simulink model "DIME12_Ctrl_dSpaceHRBMAB"  (R2018b)
settings: Solver=ode1  StartTime=0.0  StopTime=inf  FixedStep=0.5  RelTol=1e-3
PostLoadFcn:
  | if any(exist('dsrtsu_mdlpostloadfcn', 'file') ~= 0), dsrtsu_mdlpostloadfcn('Execute', bdroot); end
InitFcn:
  | , if any(exist('dsmpb_private', 'file') ~= 0), dsmpb_private('dsmpb_mdlclblib', 'Init', bdroot); end,
  | load('LUT_PSM.mat')
  | load('Torque_ts.mat')
  | 
  | p = 1;
  | L_q = 1.575e-3;
  | L_d = L_q;
  | Psi_M = 0.0353*2*pi;
  | R_s = 639e-3;
  | Ts = 1/40e3;
  | J_ges = 9.56e-5;
  | d_viskos = 0.01;
  | mpsTestMaxVelocityDmd = 166.7;
  | mpsTestVelocityDmd = 0;
  | EDC_CURRENT_CONTROL_EXECUTION_PERIOD = 4e-5;
  | 
undefined symbols (not defined in the file or in its folder): d, motor_KF, Psidq, Psiqd, q, SimSampleT
libraries: simulink x37, dsmpblib x12, simulink_extras x3
(part 1 of 2)
PreSaveFcn:
  | , if any(exist('dsmpb_private', 'file') ~= 0), dsmpb_private('dsmpb_mdlclblib', 'PreSave', bdroot); end,
CloseFcn:
  | , if any(exist('dsmpb_private', 'file') ~= 0), dsmpb_private('dsmpb_mdlclblib', 'Close', bdroot); end,
settings Model: DSMPB_ID_DATA={'3134',struct('BlockId','04db4ddd-0369-4418-ae49-28ce71638d8c','SignalIds',{{'5c51ac2c-5fbb-4ba9-aa34-33d7867766ca','a6cd89eb-b981-47d6-bc47-5ca729bc3f45','097cfed2-f50c-4e25-bc62-441cc3621ec0'}}),'3136',struct('BlockId','3590bb54-d273-4af4-9544-5048f98a2daf','SignalIds',{{'c842c855-2857-45a6-a8e5-79953c06c9eb'}}),'3137',struct('BlockId','bccae625-1341-47c7-9337-55481b633b8f','SignalIds',{{'f61f6422-2fdc-4408-804f-4fad1389e9ca'}}),'3138',struct('BlockId','34b8a974-9a5d-46c5-a0f7-f433ccad648d','SignalIds',{{'09e6ef1a-8a88-4fa6-b01f-5871e321ecb2'}}),'3139',struct('BlockId','e0cdb478-2f16-48d9-bcde-88b35d629747','SignalIds',{{'a976c208-9896-475b-afed-9b9b9f9847b2','8f7e8e4e-2c4c-4faa-aa94-dc305397ccfc','84db2b89-11f0-4bb6-8049-e2d104c4d262'}}),'3140',struct('BlockId','fd95bb8a-93e4-455d-bc68-9a6da0afcd0d','SignalIds',{{'929c58ef-2907-4469-b920-2e801e504bc2'}}),'3142',struct('BlockId','72c4edce-58e5-47fd-a414-c19eae35a3a8','SignalIds',{{'d0a6c1a2-fd8d-466a-9efe-92e242699193'}}),'3223',struct('BlockId','5770f357-64e8-43e0-9a62-efd8e5c4a994','SignalIds',{{'84e8b84b-37b0-4755-b550-56b85c125762'}}),'3326',struct('BlockId','0213ed4f-146c-4d9a-827f-511852e41879','SignalIds',{{'cdea7f12-a251-4748-b247-1d592575f419'}}),'3327',struct('BlockId','ef935bd5-43af-450c-a12d-3eb1077517d5','SignalIds',{{'a65a6045-fefa-43b6-998f-670ac0cde20a'}}),'3328',struct('BlockId','6ee705ff-6fc1-4892-a215-acc4da7c45a2','SignalIds',{{'025f1da1-06c6-4956-b1e6-82a58301fd35'}}),'3342',struct('BlockId','89047cf2-e30b-4ee5-aefe-f8c97c394358','SignalIds',{{'983c3a74-9a59-4487-a442-b115395a8b56'}})}  RTICANMMDATA=struct('GeneralSetupData',struct('modelroot','C:\Jingyuan\DIME12_HRB\SimulinkModel','generalsettings',struct('filesettings',struct('destfolder',struct('Name','RTICANMM_FILES','Check',1),'buildfolder',struct('Name','.','Check',1),'AbsDestfolder',struct('Name','C:\Jingyuan\DIME12_HRB\SimulinkModel\RTICANMM_FILES'),'AbsBuildfolder',struct('Name','C:\Jingyuan\DIME12_HRB\SimulinkModel'))),'options',struct('addpaths',1,'rmpaths',1,'addtrcexclusion',true,'cannavigator',struct('checkmonitoring',0),'show_usrtrc',0,'use_usrtrc',0),'advanced',struct('options',ones(1,100)),'MPSetup',{{}},'RTI',struct('Type','DSRT','Ver','4.2','Date','02-Nov-2019'),'modelname','DIME12_Ctrl_dSpaceHRBMAB','block','DIME12_Ctrl_dSpaceHRBMAB'))  DSRTSU_INTERNAL_RTIFPGA=150  Creator=Z0185892  LastModifiedBy=Z644053
settings DataIOCC: ReturnWorkspaceOutputs=on
settings OptimizationCC: BlockReduction=off  ConditionallyExecuteInputs=off  OptimizeBlockIOStorage=off  BufferReuse=off  GlobalBufferReuse=off  ExpressionFolding=off  LocalBlockOutputs=off  OptimizeDataStoreBuffers=off  BusAssignmentInplaceUpdate=off
settings DebuggingCC: TasksWithSamePriorityMsg=none  UnconnectedInputMsg=none  UnconnectedOutputMsg=none
settings HardwareCC: ProdBitPerPointer=32  ProdBitPerSizeT=32  ProdBitPerPtrDiffT=32  ProdLargestAtomicInteger=Integer  ProdWordSize=32  ProdHWDeviceType=Custom Processor->Custom
settings SFSimCC: MATLABDynamicMemAlloc=off
settings RTWCC: SystemTargetFile=dsrt.tlc  GenCodeOnly=on  MakeCommand=make_dsrt  TemplateMakefile=dsrt_default_tmf  Description=dSPACE Run-Time Target (for VEOS on Windows and ConfigurationDesk)  RTWVerbose=off
settings STFCustomTargetCC: TargetLangStandard=C99 (ISO)  ParMdlRefBuildCompliant=on  SystemTargetFile=dsrt.tlc
settings GRTTargetCC: CompOptLevelCompliant=off  ConcurrentExecutionCompliant=off  CombineOutputUpdateFcns=off  MatFileLogging=off  CPPClassGenCompliant=off  UseToolchainInfoCompliant=off

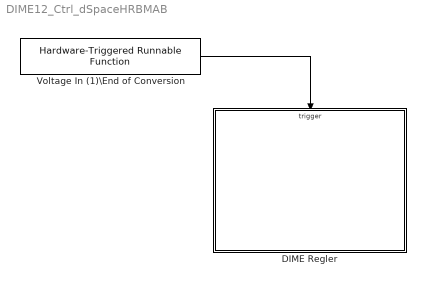
== system DIME12_Ctrl_dSpaceHRBMAB ==
  DIME Regler : Subsystem
  Voltage In (1)\End of Conversion : dsmpblib/Hardware-Triggered Runnable Function
      settings: SourceProductName=dSPACE Model Interface Blockset
  wires:
  Voltage In (1)\End of Conversion/1 -> DIME Regler/Trigger

== system DIME12_Ctrl_dSpaceHRBMAB/DIME Regler ==
  Trigger : TriggerPort  TriggerType=function-call  VariantControl=Variant  PortDimensions=1
  Bus Selector : BusSelector  OutputSignals=Omega_rps,Iphase1,Iphase2,Iphase3,Temperature
  Controller : Subsystem
  Gain : Gain  Gain=pi/30
  Outputs : Subsystem
  TqDmd : Constant  Value=2
  Velocity_RPM : Constant  Value=1000
  dSpace Measurement : Subsystem
  wires:
  TqDmd/1 -> Controller/1(TorqueDmd)
  Velocity_RPM/1 -> Gain/1
  Gain/1 -> Controller/2(VelocityDmd)
  dSpace Measurement/1(Bus Measurements) -> Bus Selector/1, Controller/3(Bus_measurements)
  Controller/1(u_alpha_beta_voltage_dmd) -> Outputs/1(AlphaBetaVoltage)
  Bus Selector/1 -> Outputs/2(meclVelocityMAB)  "<Omega_rps>"
  Bus Selector/2 -> Outputs/3(IPhase1)  "<Iphase1>"
  Bus Selector/3 -> Outputs/4(IPhase2)  "<Iphase2>"
  Bus Selector/4 -> Outputs/5(IPhase3)  "<Iphase3>"
  Bus Selector/5 -> Outputs/6(Temperature)  "<Temperature>"

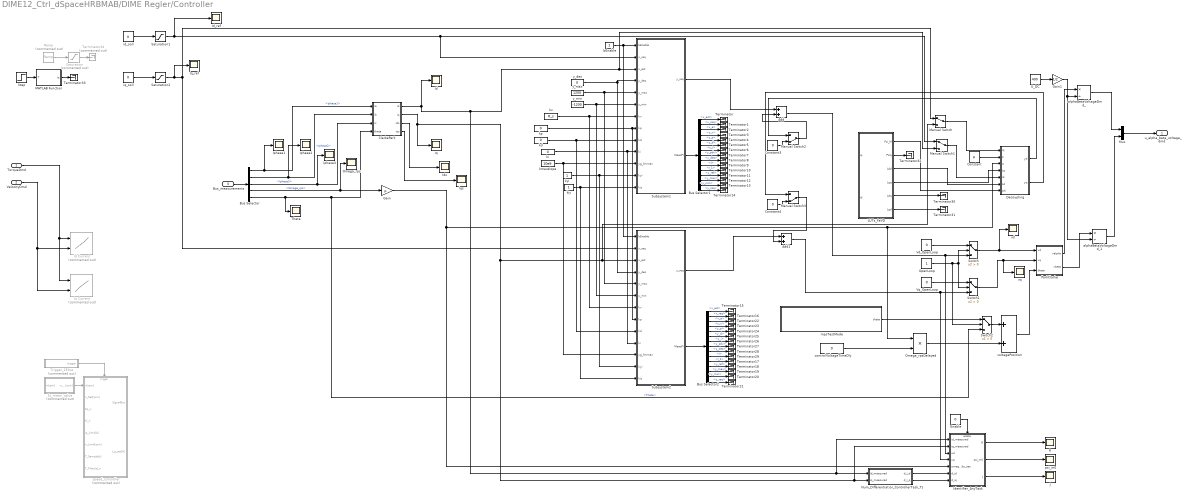
== system DIME12_Ctrl_dSpaceHRBMAB/DIME Regler/Controller ==
  TorqueDmd : Inport
  VelocityDmd : Inport  Port=2
  Bus_measurements : Inport  Port=3
  5x_mean_value : Subsystem  Commented=on
  Add : Sum
  Add1 : Sum
  Bus Selector : BusSelector  OutputSignals=Iphase1,Iphase2,Iphase3,Omega_rps,Theta
  Bus Selector1 : BusSelector  OutputSignals=x_act,x_req,x_e,y_v,y_p,y_d,y_i,y_pdv,y_des,I,I_1,y_ref,y_max,y_min,y_req
  Bus Selector2 : BusSelector  OutputSignals=x_act,x_req,x_e,y_v,y_p,y_d,y_i,y_pdv,y_des,I,I_1,y_ref,y_max,y_min,y_req
  ClarkePark : MATLAB Function  TreatAsAtomicUnit=on
  Constant : Constant  Value=p
  Constant3 : Constant  Value=0
  Constant4 : Constant  Value=0
  Decoupling : MATLAB Function  TreatAsAtomicUnit=on
  Enable : Constant  Value=0
  Gain : Gain  Gain=p
  Gain1 : Gain  Gain=1/2
  Id : Scope
  Id Current : Lookup_n-D  Commented=on  BreakpointsForDimension1=motor_KF.motTorqueDmd  BreakpointsForDimension2=motor_KF.motAbsltMeclVelocity  Table=motor_KF.idcurrent  InternalRulePriority=Speed  RndMeth=Simplest  InputSameDT=on
  Id_ref : Scope
  Identifier_AnyTask : Subsystem
  Ids : Scope
  Iphase1 : Scope
  Iphase2 : Scope
  Iphase3 : Scope
  Iq : Scope
  Iq Current : Lookup_n-D  Commented=on  BreakpointsForDimension1=motor_KF.motTorqueDmd  BreakpointsForDimension2=motor_KF.motAbsltMeclVelocity  Table=motor_KF.iqcurrent  InternalRulePriority=Speed  RndMeth=Simplest  InputSameDT=on
  Iq_ref : Scope
  Iqs : Scope
  J : Scope
  LUTs_FeVD : Subsystem
  MATLAB Function : MATLAB Function  TreatAsAtomicUnit=on
  Manual Switch : ManualSwitch
  Manual Switch1 : ManualSwitch
  Manual Switch2 : ManualSwitch  CurrentSetting=0
  Manual Switch3 : ManualSwitch  CurrentSetting=0
  Mux : Mux  Inputs=2
  Num_Differentiatior_ControllerTask_Ts : Subsystem
  Omega_rps : Scope
  Omega_rpsDelayed : Product  Inputs=**  RndMeth=Zero
  OpenLoop : Constant
  ParkClarke : MATLAB Function  TreatAsAtomicUnit=on
  R : Scope
  Ramp : simulink/Sources/Ramp  Commented=on  slope=1  start=0  InitialOutput=0
  Saturation : Saturate  Commented=on  UpperLimit=15  LowerLimit=0
  Saturation1 : Saturate  UpperLimit=18  LowerLimit=-18  LinearizeAsGain=off
  Saturation2 : Saturate  UpperLimit=18  LowerLimit=0  LinearizeAsGain=off
  Step : Step  Time=0.05  After=0
  Subsystem1 : Subsystem
  Subsystem2 : Subsystem
  Switch : Switch  Criteria=u2 > Threshold
  Switch1 : Switch  Criteria=u2 > Threshold
  Switch2 : Switch  Criteria=u2 > Threshold
  Terminator{,1..33} (34 alike) : Terminator
  Terminator34 : Terminator  Commented=on
  Theta : Scope
  Trigger_250us : Subsystem  Commented=on
  U_DC : Constant  Value=400
  Vd_OpenLoop : Constant  Value=0
  Vq_OpenLoop : Constant  Value=0
  alphaBetaVoltageDmd_ : Product  Inputs=*/  RndMeth=Zero
  alphaBetaVoltageDmd_1 : Product  Inputs=*/  RndMeth=Zero
  bEnable : Constant
  controlVoltageTimeDly : Constant  LoadFcn=|  Value=0  SampleTime=-1
      | if exist('SL_HighlightBlocks', 'file') == 2
      |     if ~SL_HighlightBlocks(gcb, [])
      |         warning(['Unable to set properties for ' gcb])
      |     end
      | end
      settings: AttributesFormatString=Changed: SampleTime
  id_soll : Constant  Value=0
  iq_soll : Constant  Value=0
  kd : Constant  Value=0
  ki : Constant  Value=0
  kiy : Constant
  kmaxslope : Constant  Value=10e9
  kp : Constant  Value=0
  kv : Constant  Value=R_s
  kyi : Constant
  mpsTestMode : Subsystem
  psi_m0 : Scope
  speed_controller : Subsystem  Commented=on
  vd : Scope
  voltagePosition : Sum
  vq : Scope
  y_des : Constant  Value=0
  y_max : Constant  Value=1200
  y_min : Constant  Value=-1200
  u_alpha_beta_voltage_dmd : Outport  VectorParamsAs1DForOutWhenUnconnected=on
  wires:
  TorqueDmd/1 -> Iq Current/1, Id Current/1
  VelocityDmd/1 -> Iq Current/2, Id Current/2
  Bus Selector/2 -> Iphase2/1, ClarkePark/2(ib)  "<Iphase2>"
  Bus Selector/1 -> Iphase1/1, ClarkePark/1(ia)  "<Iphase1>"
  Bus Selector/3 -> Iphase3/1, ClarkePark/3(ic)  "<Iphase3>"
  Bus_measurements/1 -> Bus Selector/1
  Bus Selector/4 -> Gain/1, Omega_rps/1  "<Omega_rps>"
  Bus Selector1/9 -> Terminator8/1  "<y_des>"
  Bus Selector1/6 -> Terminator5/1  "<y_d>"
  Bus Selector1/12 -> Terminator11/1  "<y_ref>"
  Bus Selector1/15 -> Terminator14/1  "<y_req>"
  kp/1 -> Subsystem2/8(kp), Subsystem1/8(kp)
  Bus Selector1/4 -> Terminator3/1  "<y_v>"
  Bus Selector1/5 -> Terminator4/1  "<y_p>"
  Bus Selector1/2 -> Terminator1/1  "<x_req>"
  Bus Selector1/13 -> Terminator12/1  "<y_max>"
  kd/1 -> Subsystem2/9(kd), Subsystem1/9(kd)
  Bus Selector1/8 -> Terminator7/1  "<y_pdv>"
  Bus Selector1/10 -> Terminator9/1  "<I>"
  Subsystem1/2(MeasPi) -> Bus Selector1/1
  Bus Selector1/7 -> Terminator6/1  "<y_i>"
  Bus Selector1/1 -> Terminator/1  "<x_act>"
  Bus Selector1/14 -> Terminator13/1  "<y_min>"
  Bus Selector1/11 -> Terminator10/1  "<I_1>"
  Bus Selector1/3 -> Terminator2/1  "<x_e>"
  Bus Selector2/9 -> Terminator28/1  "<y_des>"
  y_des/1 -> Subsystem1/4(y_des), Subsystem2/4(y_des)
  kmaxslope/1 -> Subsystem2/11(yg_limmax), Subsystem1/11(yg_limmax)
  kiy/1 -> Subsystem2/13(kiy), Subsystem1/13(kiy)
  y_max/1 -> Subsystem2/5(y_max), Subsystem1/5(y_max)
  Bus Selector2/6 -> Terminator25/1  "<y_d>"
  Bus Selector2/12 -> Terminator18/1  "<y_ref>"
  y_min/1 -> Subsystem2/6(y_min), Subsystem1/6(y_min)
  Bus Selector2/15 -> Terminator21/1  "<y_req>"
  Bus Selector2/4 -> Terminator23/1  "<y_v>"
  Bus Selector2/5 -> Terminator24/1  "<y_p>"
  Bus Selector2/2 -> Terminator16/1  "<x_req>"
  Bus Selector2/13 -> Terminator19/1  "<y_max>"
  ki/1 -> Subsystem2/10(ki), Subsystem1/10(ki)
  kyi/1 -> Subsystem1/12(kyi), Subsystem2/12(kyi)
  kv/1 -> Subsystem2/7(kv), Subsystem1/7(kv)
  Bus Selector2/8 -> Terminator27/1  "<y_pdv>"
  Bus Selector2/10 -> Terminator29/1  "<I>"
  Subsystem2/2(MeasPi) -> Bus Selector2/1
  Bus Selector2/7 -> Terminator26/1  "<y_i>"
  Bus Selector2/1 -> Terminator15/1  "<x_act>"
  Bus Selector2/14 -> Terminator20/1  "<y_min>"
  Bus Selector2/11 -> Terminator17/1  "<I_1>"
  Bus Selector2/3 -> Terminator22/1  "<x_e>"
  bEnable/1 -> Subsystem2/1(bEnable), Subsystem1/1(bEnable)
  ClarkePark/1(id) -> Identifier_AnyTask/1(id_measured), Num_Differentiatior_ControllerTask_Ts/1(id_measured), Manual Switch1/2, Subsystem1/3(x_act), Id/1
  ClarkePark/2(iq) -> Iq/1, Identifier_AnyTask/2(iq_measured), Num_Differentiatior_ControllerTask_Ts/2(iq_measured), Manual Switch/2, Subsystem2/3(x_act)
  Subsystem1/1(y_req) -> Add/1
  Decoupling/1(yd) -> Manual Switch2/1
  Subsystem2/1(y_req) -> Add1/1
  Decoupling/2(yq) -> Manual Switch3/1
  Add1/1 -> Identifier_AnyTask/4(uq), Switch1/3
  Add/1 -> Identifier_AnyTask/3(ud), Switch/3
  LUTs_FeVD/6(Lqd) -> Terminator31/1
  LUTs_FeVD/5(Ldq) -> Terminator30/1
  LUTs_FeVD/3(Ldd) -> Decoupling/6(Ld)
  LUTs_FeVD/4(Lqq) -> Decoupling/4(Lq)
  LUTs_FeVD/1(Psi_M) -> Decoupling/7(phi)
  Constant/1 -> Decoupling/2(p)
  Gain/1 -> Identifier_AnyTask/5(omega_elec_1by_sec), Omega_rpsDelayed/1, Decoupling/3(w)
  LUTs_FeVD/2(Psiq) -> Terminator32/1
  ParkClarke/1(valpha) -> alphaBetaVoltageDmd_/1
  U_DC/1 -> Gain1/1
  ParkClarke/2(vbeta) -> alphaBetaVoltageDmd_1/1
  alphaBetaVoltageDmd_/1 -> Mux/1
  alphaBetaVoltageDmd_1/1 -> Mux/2
  Mux/1 -> u_alpha_beta_voltage_dmd/1
  id_soll/1 -> Saturation1/1
  iq_soll/1 -> Saturation2/1
  Manual Switch/1 -> Decoupling/1(iq)
  Manual Switch1/1 -> Decoupling/5(id)
  Constant3/1 -> Manual Switch2/2
  Manual Switch2/1 -> Add/2
  Constant4/1 -> Manual Switch3/2
  Manual Switch3/1 -> Add1/2
  Step/1 -> MATLAB Function/1(T)
  Bus Selector/5 -> Theta/1, Switch2/3, ClarkePark/4(theta)  "<Theta>"
  Vd_OpenLoop/1 -> Switch/1
  Switch/1 -> vd/1, ParkClarke/1(vd)
  Vq_OpenLoop/1 -> Switch1/1
  Switch1/1 -> vq/1, ParkClarke/2(vq)
  mpsTestMode/1(theta) -> Switch2/1
  OpenLoop/1 -> Switch2/2, Switch/2, Switch1/2
  Switch2/1 -> voltagePosition/1
  MATLAB Function/1(iq) -> Terminator33/1
  controlVoltageTimeDly/1 -> Omega_rpsDelayed/2
  Omega_rpsDelayed/1 -> voltagePosition/2
  voltagePosition/1 -> ParkClarke/3(theta)
  Ramp/1 -> Saturation/1
  Saturation/1 -> Terminator34/1
  Saturation1/1 -> Id_ref/1, Manual Switch1/1, Subsystem1/2(x_req)
  Saturation2/1 -> Iq_ref/1, Manual Switch/1, Subsystem2/2(x_req)
  ClarkePark/3(ids) -> Ids/1
  ClarkePark/4(iqs) -> Iqs/1
  Num_Differentiatior_ControllerTask_Ts/1(d_i_d) -> Identifier_AnyTask/6(d_id)
  Identifier_AnyTask/2(psi_m0) -> psi_m0/1
  Identifier_AnyTask/3(J) -> J/1
  Num_Differentiatior_ControllerTask_Ts/2(d_i_q) -> Identifier_AnyTask/7(d_iq)
  Identifier_AnyTask/1(R) -> R/1
  Enable/1 -> Identifier_AnyTask/Enable
  Gain1/1 -> alphaBetaVoltageDmd_/2, alphaBetaVoltageDmd_1/2
  5x_mean_value/1(n_mean[rpm]) -> speed_controller/1(n[rpm])
  Trigger_250us/1(trigger) -> speed_controller/Trigger

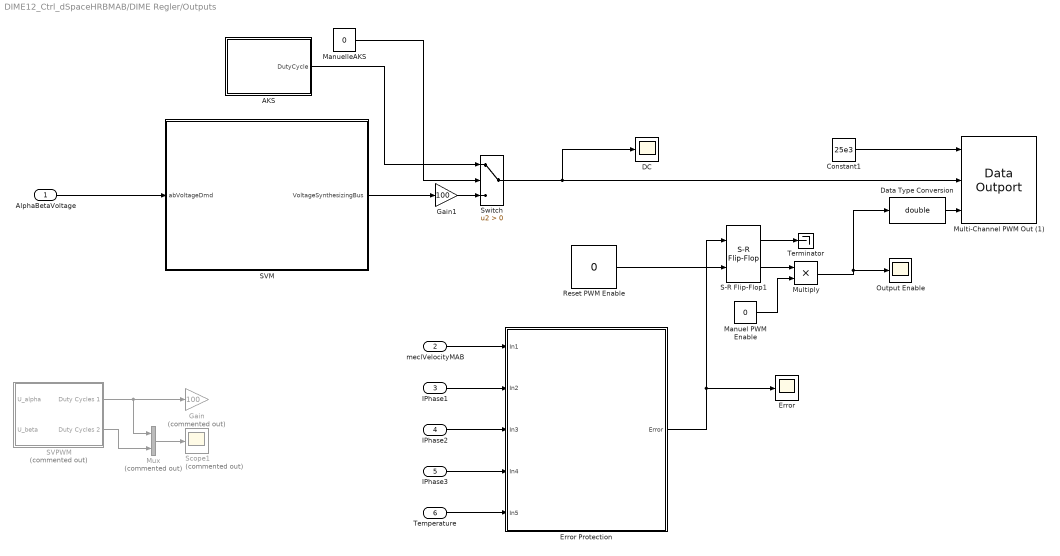
== system DIME12_Ctrl_dSpaceHRBMAB/DIME Regler/Outputs ==
  AlphaBetaVoltage : Inport
  meclVelocityMAB : Inport  Port=2
  IPhase1 : Inport  Port=3
  IPhase2 : Inport  Port=4
  IPhase3 : Inport  Port=5
  Temperature : Inport  Port=6
  AKS : Subsystem
  Constant1 : Constant  Value=25e3
  DC : Scope
  Data Type Conversion : DataTypeConversion  OutDataTypeStr=double
  Error : Scope
  Error Protection : Subsystem
  Gain : Gain  Commented=on  Gain=100
  Gain1 : Gain  Gain=100
  Manuel PWM Enable : Constant  Value=0
  ManuelleAKS : Constant  Value=0
  Multi-Channel PWM Out (1) : dsmpblib/Data Outport  Priority=-10000
      settings: SourceProductName=dSPACE Model Interface Blockset
  Multiply : Product
  Mux : Mux  Commented=on  Inputs=2
  Output Enable : Scope
  Reset PWM Enable : Constant  Value=0  OutDataTypeStr=Inherit: Inherit via back propagation
  S-R Flip-Flop1 : simulink_extras/Flip Flops/S-R Flip-Flop  initial_condition=1
  SVM : Subsystem  VariantControl=Variant
  SVPWM : Subsystem  Commented=on
  Scope1 : Scope  Commented=on
  Switch : Switch  Criteria=u2 > Threshold
  Terminator : Terminator
  wires:
  Constant1/1 -> Multi-Channel PWM Out (1)/1
  SVPWM/2(Duty Cycles 2) -> Mux/2
  SVPWM/1(Duty Cycles 1) -> Mux/1, Gain/1
  Mux/1 -> Scope1/1
  AlphaBetaVoltage/1 -> SVM/1(abVoltageDmd)
  SVM/1(VoltageSynthesizingBus) -> Gain1/1
  AKS/1(DutyCycle) -> Switch/1
  ManuelleAKS/1 -> Switch/2
  Gain1/1 -> Switch/3
  Reset PWM Enable/1 -> S-R Flip-Flop1/2
  meclVelocityMAB/1 -> Error Protection/1(In1)
  IPhase1/1 -> Error Protection/2(In2)
  IPhase2/1 -> Error Protection/3(In3)
  IPhase3/1 -> Error Protection/4(In4)
  Temperature/1 -> Error Protection/5(In5)
  Error Protection/1(Error) -> S-R Flip-Flop1/1, Error/1
  S-R Flip-Flop1/1 -> Terminator/1
  Data Type Conversion/1 -> Multi-Channel PWM Out (1)/3
  S-R Flip-Flop1/2 -> Multiply/1
  Manuel PWM Enable/1 -> Multiply/2
  Multiply/1 -> Output Enable/1, Data Type Conversion/1
  Switch/1 -> Multi-Channel PWM Out (1)/2, DC/1

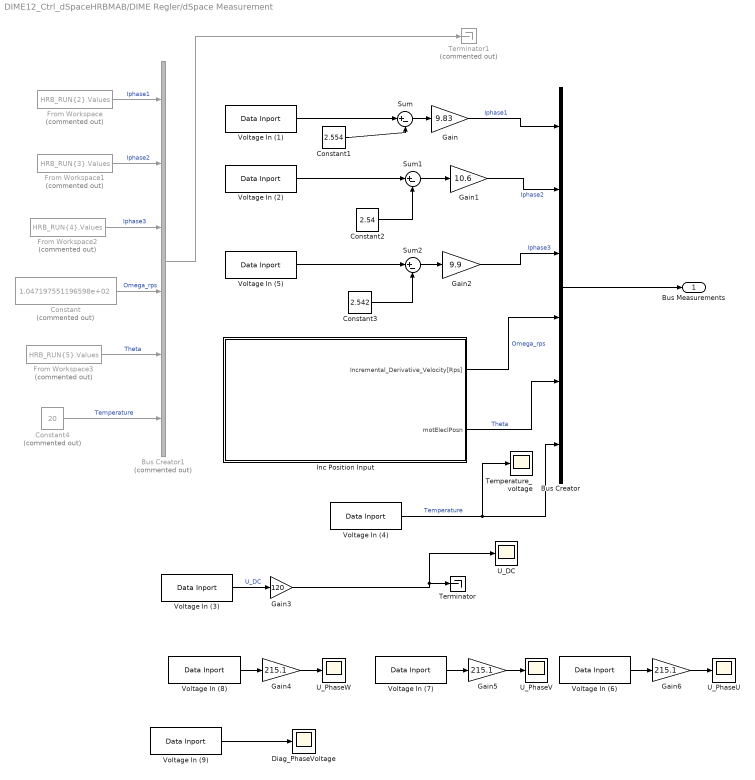
== system DIME12_Ctrl_dSpaceHRBMAB/DIME Regler/dSpace Measurement ==
  Bus Creator : BusCreator  Inputs=6
  Bus Creator1 : BusCreator  Commented=on  Inputs=6
  Constant : Constant  Commented=on  Value=1.047197551196598e+02  SampleTime=-1
  Constant1 : Constant  Value=2.554
  Constant2 : Constant  Value=2.54
  Constant3 : Constant  Value=2.542
  Constant4 : Constant  Commented=on  Value=20  SampleTime=-1
  Diag_PhaseVoltage : Scope
  From Workspace : FromWorkspace  Commented=on  VariableName=HRB_RUN{2}.Values
  From Workspace1 : FromWorkspace  Commented=on  VariableName=HRB_RUN{3}.Values
  From Workspace2 : FromWorkspace  Commented=on  VariableName=HRB_RUN{4}.Values
  From Workspace3 : FromWorkspace  Commented=on  VariableName=HRB_RUN{5}.Values
  Gain : Gain  Gain=9.83
  Gain1 : Gain  Gain=10.6
  Gain2 : Gain  Gain=9.9
  Gain3 : Gain  Gain=120
  Gain4 : Gain  Gain=215.1
  Gain5 : Gain  Gain=215.1
  Gain6 : Gain  Gain=215.1
  Inc Position Input : Subsystem
  Sum : Sum  Inputs=|+-
  Sum1 : Sum  Inputs=|+-
  Sum2 : Sum  Inputs=|+-
  Temperature_voltage : Scope
  Terminator : Terminator
  Terminator1 : Terminator  Commented=on
  U_DC : Scope
  U_PhaseU : Scope
  U_PhaseV : Scope
  U_PhaseW : Scope
  Voltage In (1) : dsmpblib/Data Inport  Priority=10000
      settings: SourceProductName=dSPACE Model Interface Blockset
  Voltage In (2) : dsmpblib/Data Inport  Priority=10000
      settings: SourceProductName=dSPACE Model Interface Blockset
  Voltage In (3) : dsmpblib/Data Inport  Priority=10000
      settings: SourceProductName=dSPACE Model Interface Blockset
  Voltage In (4) : dsmpblib/Data Inport  Priority=10000
      settings: SourceProductName=dSPACE Model Interface Blockset
  Voltage In (5) : dsmpblib/Data Inport  Priority=10000
      settings: SourceProductName=dSPACE Model Interface Blockset
  Voltage In (6) : dsmpblib/Data Inport  Priority=10000
      settings: SourceProductName=dSPACE Model Interface Blockset
  Voltage In (7) : dsmpblib/Data Inport  Priority=10000
      settings: SourceProductName=dSPACE Model Interface Blockset
  Voltage In (8) : dsmpblib/Data Inport  Priority=10000
      settings: SourceProductName=dSPACE Model Interface Blockset
  Voltage In (9) : dsmpblib/Data Inport  Priority=10000
      settings: SourceProductName=dSPACE Model Interface Blockset
  Bus Measurements : Outport
  wires:
  Constant2/1 -> Sum1/2
  Sum1/1 -> Gain1/1
  Gain1/1 -> Bus Creator/2  "Iphase2"
  Voltage In (1)/1 -> Sum/1
  Voltage In (5)/1 -> Sum2/1
  Gain/1 -> Bus Creator/1  "Iphase1"
  Sum2/1 -> Gain2/1
  Voltage In (2)/1 -> Sum1/1
  Constant1/1 -> Sum/2
  Gain2/1 -> Bus Creator/3  "Iphase3"
  Constant3/1 -> Sum2/2
  Sum/1 -> Gain/1
  Inc Position Input/1(Incremental_Derivative_Velocity[Rps]) -> Bus Creator/4  "Omega_rps"
  Inc Position Input/2(motEleclPosn) -> Bus Creator/5  "Theta"
  Voltage In (4)/1 -> Temperature_voltage/1, Bus Creator/6  "Temperature"
  From Workspace2/1 -> Bus Creator1/3  "Iphase3"
  From Workspace3/1 -> Bus Creator1/5  "Theta"
  Constant/1 -> Bus Creator1/4  "Omega_rps"
  Constant4/1 -> Bus Creator1/6  "Temperature"
  Voltage In (3)/1 -> Gain3/1  "U_DC"
  Gain3/1 -> U_DC/1, Terminator/1
  From Workspace/1 -> Bus Creator1/1  "Iphase1"
  From Workspace1/1 -> Bus Creator1/2  "Iphase2"
  Bus Creator1/1 -> Terminator1/1
  Bus Creator/1 -> Bus Measurements/1
  Voltage In (8)/1 -> Gain4/1
  Voltage In (7)/1 -> Gain5/1
  Voltage In (6)/1 -> Gain6/1
  Gain4/1 -> U_PhaseW/1
  Gain5/1 -> U_PhaseV/1
  Gain6/1 -> U_PhaseU/1
  Voltage In (9)/1 -> Diag_PhaseVoltage/1

== system DIME12_Ctrl_dSpaceHRBMAB/DIME Regler/Controller/5x_mean_value ==
  n[rpm] : Inport
  Gain : Gain  Gain=1/5
  Memory{,1..3} (4 alike) : Memory  InheritSampleTime=on
  Sum : Sum  Inputs=+++++
  n_mean[rpm] : Outport
  wires:
  n[rpm]/1 -> Sum/1, Memory/1
  Memory/1 -> Sum/2, Memory1/1
  Memory1/1 -> Sum/3, Memory2/1
  Memory2/1 -> Sum/4, Memory3/1
  Memory3/1 -> Sum/5
  Sum/1 -> Gain/1
  Gain/1 -> n_mean[rpm]/1

== system DIME12_Ctrl_dSpaceHRBMAB/DIME Regler/Controller/Identifier_AnyTask ==
  id_measured : Inport
  iq_measured : Inport  Port=2
  ud : Inport  Port=3
  uq : Inport  Port=4
  omega_elec_1by_sec : Inport  Port=5
  d_id : Inport  Port=6
  d_iq : Inport  Port=7
  Enable : EnablePort  StatesWhenEnabling=reset
  NN Identifier : MATLAB Function  TreatAsAtomicUnit=on
  StepsizeIntegrator : Constant  Value=1e-4
  gains : Constant  Value=1e-3
  psim0_est : Constant  Value=0.1
  takeover : Constant  Value=0
  R : Outport  VectorParamsAs1DForOutWhenUnconnected=on
  psi_m0 : Outport  Port=2  VectorParamsAs1DForOutWhenUnconnected=on
  J : Outport  Port=3  VectorParamsAs1DForOutWhenUnconnected=on
  wires:
  id_measured/1 -> NN Identifier/2(id)
  StepsizeIntegrator/1 -> NN Identifier/1(h)
  gains/1 -> NN Identifier/12(Gamma_W_psi), NN Identifier/11(Gamma_Theta_psi), NN Identifier/10(Gamma_W_R), NN Identifier/9(Gamma_Theta_R)
  NN Identifier/2(psi_m0) -> psi_m0/1
  NN Identifier/1(R) -> R/1
  NN Identifier/3(J) -> J/1
  uq/1 -> NN Identifier/5(uq)
  omega_elec_1by_sec/1 -> NN Identifier/6(omega)
  ud/1 -> NN Identifier/4(ud)
  iq_measured/1 -> NN Identifier/3(iq)
  d_id/1 -> NN Identifier/7(d_id)
  d_iq/1 -> NN Identifier/8(d_iq)
  takeover/1 -> NN Identifier/13(takeover)
  psim0_est/1 -> NN Identifier/14(psim0_est)

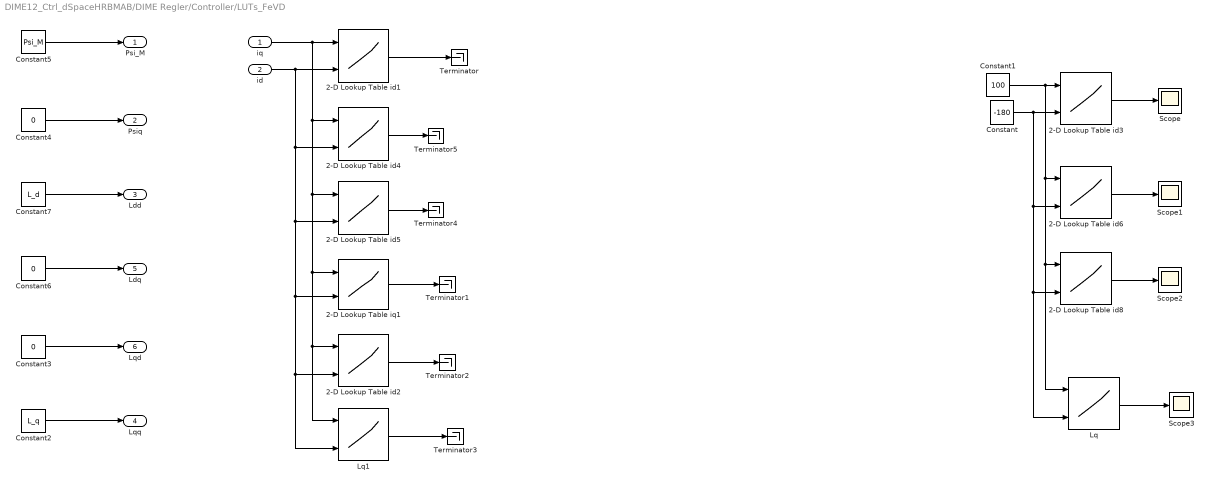
== system DIME12_Ctrl_dSpaceHRBMAB/DIME Regler/Controller/LUTs_FeVD ==
  iq : Inport
  id : Inport  Port=2
  2-D Lookup Table id1 : Lookup_n-D  BreakpointsForDimension1=|  BreakpointsForDimension2=|  Table=motor_KF.Psi_d'  InternalRulePriority=Speed  RndMeth=Simplest  InputSameDT=on
      BreakpointsForDimension2=|
      | [-220
      | -200
      | -180
      | -160
      | -140
      | -120
      | -100
      | -80
      | -60
      | -40
      | -20
      | 0
      | ]
      BreakpointsForDimension1=|
      | [0	20	40	60	80	100	120	140	160	180	200	220
      | ]
  2-D Lookup Table id2 : Lookup_n-D  BreakpointsForDimension1=q  BreakpointsForDimension2=d  Table=Psiqd  InternalRulePriority=Speed  RndMeth=Simplest  InputSameDT=on
  2-D Lookup Table id3 : Lookup_n-D  BreakpointsForDimension1=|  BreakpointsForDimension2=|  Table=motor_KF.Psi_d'  InternalRulePriority=Speed  RndMeth=Simplest  InputSameDT=on
      BreakpointsForDimension2=|
      | [-220
      | -200
      | -180
      | -160
      | -140
      | -120
      | -100
      | -80
      | -60
      | -40
      | -20
      | 0
      | ]
      BreakpointsForDimension1=|
      | [0	20	40	60	80	100	120	140	160	180	200	220
      | ]
  2-D Lookup Table id4 : Lookup_n-D  BreakpointsForDimension1=motor_KF.iqgrid  BreakpointsForDimension2=motor_KF.idgrid  Table=motor_KF.Psi_q'  InternalRulePriority=Speed  RndMeth=Simplest  InputSameDT=on
  2-D Lookup Table id5 : Lookup_n-D  BreakpointsForDimension1=motor_KF.iqgrid  BreakpointsForDimension2=motor_KF.idgrid  Table=motor_KF.Ld'  InternalRulePriority=Speed  RndMeth=Simplest  InputSameDT=on
  2-D Lookup Table id6 : Lookup_n-D  BreakpointsForDimension1=motor_KF.iqgrid  BreakpointsForDimension2=motor_KF.idgrid  Table=motor_KF.Psi_q'  InternalRulePriority=Speed  RndMeth=Simplest  InputSameDT=on
  2-D Lookup Table id8 : Lookup_n-D  BreakpointsForDimension1=motor_KF.iqgrid  BreakpointsForDimension2=motor_KF.idgrid  Table=motor_KF.Ld'  InternalRulePriority=Speed  RndMeth=Simplest  InputSameDT=on
  2-D Lookup Table iq1 : Lookup_n-D  BreakpointsForDimension1=q  BreakpointsForDimension2=d  Table=Psidq  InternalRulePriority=Speed  RndMeth=Simplest  InputSameDT=on
  Constant : Constant  Value=-180
  Constant1 : Constant  Value=100
  Constant2 : Constant  Value=L_q
  Constant3 : Constant  Value=0
  Constant4 : Constant  Value=0
  Constant5 : Constant  Value=Psi_M
  Constant6 : Constant  Value=0
  Constant7 : Constant  Value=L_d
  Lq : Lookup_n-D  BreakpointsForDimension1=motor_KF.iqgrid  BreakpointsForDimension2=motor_KF.idgrid  Table=motor_KF.Lq'  InternalRulePriority=Speed  RndMeth=Simplest  InputSameDT=on
  Lq1 : Lookup_n-D  BreakpointsForDimension1=motor_KF.iqgrid  BreakpointsForDimension2=motor_KF.idgrid  Table=motor_KF.Lq'  InternalRulePriority=Speed  RndMeth=Simplest  InputSameDT=on
  Scope{,1..3} (4 alike) : Scope
  Terminator{,1..5} (6 alike) : Terminator
  Psi_M : Outport  VectorParamsAs1DForOutWhenUnconnected=on
  Psiq : Outport  Port=2  VectorParamsAs1DForOutWhenUnconnected=on
  Ldd : Outport  Port=3  VectorParamsAs1DForOutWhenUnconnected=on
  Lqq : Outport  Port=4  VectorParamsAs1DForOutWhenUnconnected=on
  Ldq : Outport  Port=5  VectorParamsAs1DForOutWhenUnconnected=on
  Lqd : Outport  Port=6  VectorParamsAs1DForOutWhenUnconnected=on
  wires:
  iq/1 -> 2-D Lookup Table id1/1, 2-D Lookup Table id4/1, 2-D Lookup Table id5/1, Lq1/1, 2-D Lookup Table id2/1, 2-D Lookup Table iq1/1
  id/1 -> 2-D Lookup Table id1/2, 2-D Lookup Table id4/2, 2-D Lookup Table id5/2, Lq1/2, 2-D Lookup Table id2/2, 2-D Lookup Table iq1/2
  2-D Lookup Table id3/1 -> Scope/1
  Constant1/1 -> Lq/1, 2-D Lookup Table id8/1, 2-D Lookup Table id6/1, 2-D Lookup Table id3/1
  Constant/1 -> Lq/2, 2-D Lookup Table id8/2, 2-D Lookup Table id6/2, 2-D Lookup Table id3/2
  2-D Lookup Table id6/1 -> Scope1/1
  Lq/1 -> Scope3/1
  2-D Lookup Table id8/1 -> Scope2/1
  Constant4/1 -> Psiq/1
  Constant5/1 -> Psi_M/1
  Constant3/1 -> Lqd/1
  Constant7/1 -> Ldd/1
  Constant2/1 -> Lqq/1
  Constant6/1 -> Ldq/1
  2-D Lookup Table id1/1 -> Terminator/1
  Lq1/1 -> Terminator3/1
  2-D Lookup Table id2/1 -> Terminator2/1
  2-D Lookup Table iq1/1 -> Terminator1/1
  2-D Lookup Table id5/1 -> Terminator4/1
  2-D Lookup Table id4/1 -> Terminator5/1

== system DIME12_Ctrl_dSpaceHRBMAB/DIME Regler/Controller/Num_Differentiatior_ControllerTask_Ts ==
  id_measured : Inport
  iq_measured : Inport  Port=2
  Diff_Gain : Gain  Gain=5e3
  Diff_Gain2 : Gain  Gain=5e3
  Int : Subsystem
  Int1 : Subsystem
  Sum : Sum  Inputs=|+-
  Sum1 : Sum  Inputs=|+-
  compare_id : Scope  NumInputPorts=2
  compare_iq : Scope  NumInputPorts=2
  d_i_d : Outport  VectorParamsAs1DForOutWhenUnconnected=on
  d_i_q : Outport  Port=2  VectorParamsAs1DForOutWhenUnconnected=on
  wires:
  Sum/1 -> Diff_Gain/1
  Diff_Gain2/1 -> d_i_q/1, Int1/1(i_q_p)
  Diff_Gain/1 -> d_i_d/1, Int/1(i_d_p)
  Int/1(i_d) -> compare_id/2, Sum/2  "id"
  Sum1/1 -> Diff_Gain2/1
  Int1/1(i_q) -> compare_iq/2, Sum1/2  "iq"
  id_measured/1 -> compare_id/1, Sum/1
  iq_measured/1 -> compare_iq/1, Sum1/1

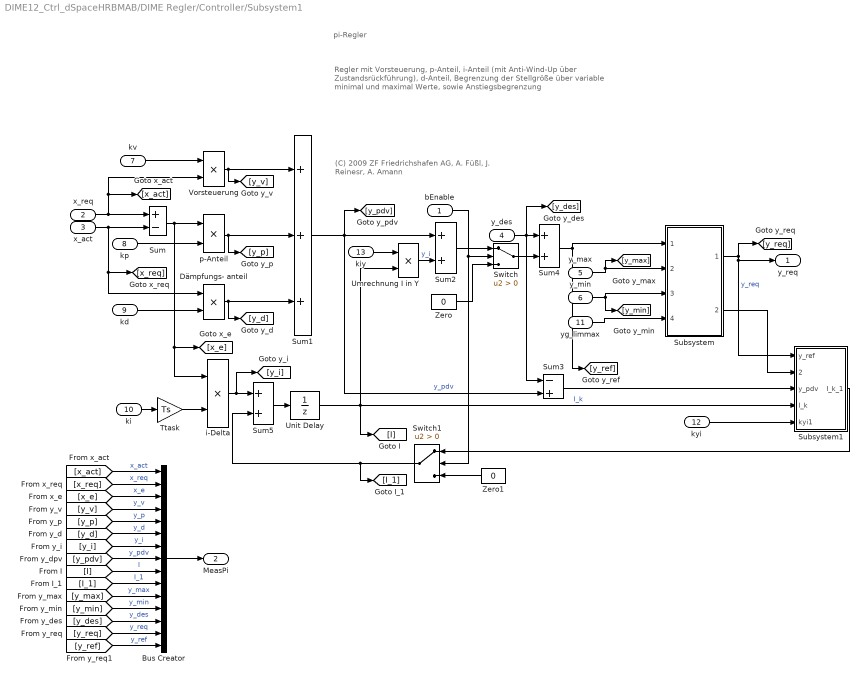
== system DIME12_Ctrl_dSpaceHRBMAB/DIME Regler/Controller/Subsystem1 ==
  note: Regler mit Vorsteuerung,
      | p-Anteil,
      | i-Anteil (mit Anti-Wind-Up über Zustandsrückführung),
      | d-Anteil,
      | Begrenzung der Stellgröße über
      | variable minimal und maximal Werte,
      | sowie Anstiegsbegrenzung
  note: pi-Regler
  note: (C) 2009 ZF Friedrichshafen AG,
      | A. Füßl, J. Reinesr, A. Amann
  bEnable : Inport
  x_req : Inport  Port=2
  x_act : Inport  Port=3
  y_des : Inport  Port=4
  y_max : Inport  Port=5
  y_min : Inport  Port=6
  kv : Inport  Port=7
  kp : Inport  Port=8
  kd : Inport  Port=9
  ki : Inport  Port=10
  yg_limmax : Inport  Port=11
  kyi : Inport  Port=12
  kiy : Inport  Port=13
  Bus Creator : BusCreator  Inputs=15
  Dämpfungs- anteil : Product  SaturateOnIntegerOverflow=on  OutDataTypeStr=Inherit: Same as first input
  Subsystem : Subsystem
  Subsystem1 : Subsystem
  Sum : Sum  Inputs=+-  SaturateOnIntegerOverflow=on
  Sum1 : Sum  Inputs=+++  SaturateOnIntegerOverflow=on
  Sum2 : Sum  SaturateOnIntegerOverflow=on
  Sum3 : Sum  Inputs=-+  SaturateOnIntegerOverflow=on
  Sum4 : Sum  SaturateOnIntegerOverflow=on
  Sum5 : Sum  SaturateOnIntegerOverflow=on
  Switch : Switch  Criteria=u2 > Threshold
  Switch1 : Switch  Criteria=u2 > Threshold
  Ttask : Gain  Gain=Ts  SaturateOnIntegerOverflow=on  OutDataTypeStr=Inherit: Same as input  ParamDataTypeStr=Inherit: Same as input
  Umrechnung I in Y : Product  SaturateOnIntegerOverflow=on  OutDataTypeStr=Inherit: Same as first input
  Unit Delay : UnitDelay  SampleTime=-1
  Vorsteuerung : Product  SaturateOnIntegerOverflow=on  OutDataTypeStr=Inherit: Same as first input
  Zero : Constant  Value=0
  Zero1 : Constant  Value=0
  i-Delta : Product  SaturateOnIntegerOverflow=on  OutDataTypeStr=Inherit: Same as first input
  p-Anteil : Product  SaturateOnIntegerOverflow=on  OutDataTypeStr=Inherit: Same as first input
  y_req : Outport
  MeasPi : Outport  Port=2
  wires:
  [y_d] -> Bus Creator/6  "y_d"
  kp/1 -> p-Anteil/2
  x_req/1 -> Vorsteuerung/2, [x_act], Sum/1
  yg_limmax/1 -> Subsystem/4(yg_limmax1)
  [y_req] -> Bus Creator/14  "y_req"
  p-Anteil/1 -> [y_p], Sum1/2
  y_des/1 -> Sum3/1, Sum4/1, [y_des]
  Subsystem/1(y_req1) -> Subsystem1/1(y_ref), y_req/1, [y_req]  "y_req"
  Switch1/1 -> [I_1], Sum5/2
  kyi/1 -> Subsystem1/5(kyi1)
  Subsystem1/1(I_k_1) -> Switch1/1
  [y_i] -> Bus Creator/7  "y_i"
  y_max/1 -> Subsystem/2(y_max1), [y_max]
  y_min/1 -> Subsystem/3(y_min1), [y_min]
  x_act/1 -> Dämpfungs- anteil/1, [x_req], Sum/2
  Sum4/1 -> Subsystem/1(x_act1), [y_ref]
  Switch/1 -> Sum4/2
  Umrechnung I in Y/1 -> Sum2/2  "y_i"
  Subsystem/2(ydif_lim) -> Subsystem1/2(ydif_lim)
  [y_max] -> Bus Creator/11  "y_max"
  [y_pdv] -> Bus Creator/8  "y_pdv"
  Sum1/1 -> Sum3/2, [y_pdv], Sum2/1  "y_pdv"
  [y_p] -> Bus Creator/5  "y_p"
  Sum/1 -> p-Anteil/1, [x_e], i-Delta/1
  Vorsteuerung/1 -> [y_v], Sum1/1
  [y_des] -> Bus Creator/13  "y_des"
  Dämpfungs- anteil/1 -> [y_d], Sum1/3
  Sum2/1 -> Switch/1
  [y_v] -> Bus Creator/4  "y_v"
  [I_1] -> Bus Creator/10  "I_1"
  kiy/1 -> Umrechnung I in Y/1
  Sum5/1 -> Unit Delay/1
  kv/1 -> Vorsteuerung/1
  [I] -> Bus Creator/9  "I"
  [x_act] -> Bus Creator/1  "x_act"
  Unit Delay/1 -> Subsystem1/4(I_k), Umrechnung I in Y/2, [I]  "I_k"
  [y_min] -> Bus Creator/12  "y_min"
  [x_e] -> Bus Creator/3  "x_e"
  Ttask/1 -> i-Delta/2
  kd/1 -> Dämpfungs- anteil/2
  ki/1 -> Ttask/1
  [x_req] -> Bus Creator/2  "x_req"
  Sum3/1 -> Subsystem1/3(y_pdv)
  Bus Creator/1 -> MeasPi/1
  [y_ref] -> Bus Creator/15  "y_ref"
  bEnable/1 -> Switch1/2, Switch/2
  Zero/1 -> Switch/3
  Zero1/1 -> Switch1/3
  i-Delta/1 -> [y_i], Sum5/1

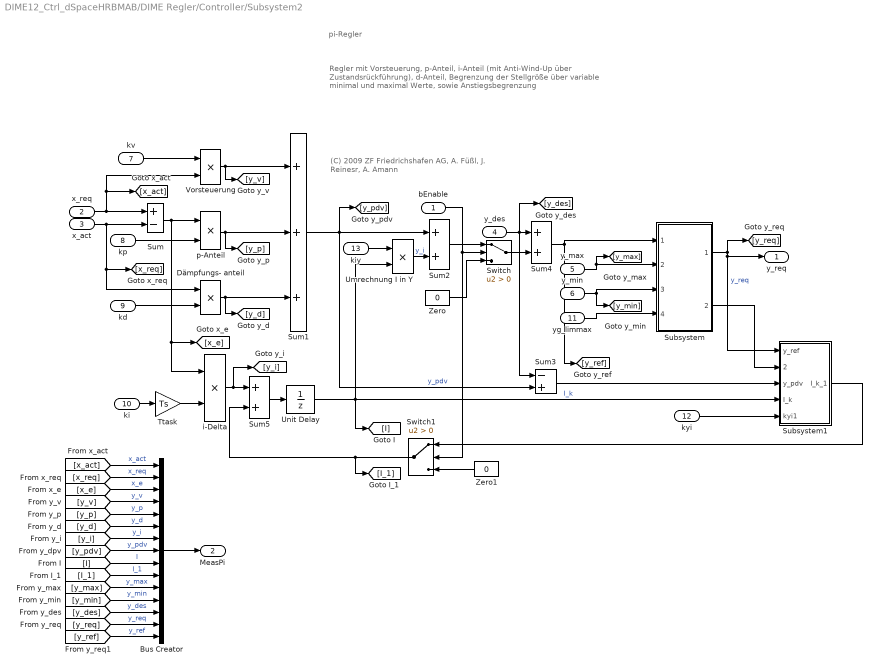
== system DIME12_Ctrl_dSpaceHRBMAB/DIME Regler/Controller/Subsystem2 ==
  note: Regler mit Vorsteuerung,
      | p-Anteil,
      | i-Anteil (mit Anti-Wind-Up über Zustandsrückführung),
      | d-Anteil,
      | Begrenzung der Stellgröße über
      | variable minimal und maximal Werte,
      | sowie Anstiegsbegrenzung
  note: pi-Regler
  note: (C) 2009 ZF Friedrichshafen AG,
      | A. Füßl, J. Reinesr, A. Amann
  bEnable : Inport
  x_req : Inport  Port=2
  x_act : Inport  Port=3
  y_des : Inport  Port=4
  y_max : Inport  Port=5
  y_min : Inport  Port=6
  kv : Inport  Port=7
  kp : Inport  Port=8
  kd : Inport  Port=9
  ki : Inport  Port=10
  yg_limmax : Inport  Port=11
  kyi : Inport  Port=12
  kiy : Inport  Port=13
  Bus Creator : BusCreator  Inputs=15
  Dämpfungs- anteil : Product  SaturateOnIntegerOverflow=on  OutDataTypeStr=Inherit: Same as first input
  Subsystem : Subsystem
  Subsystem1 : Subsystem
  Sum : Sum  Inputs=+-  SaturateOnIntegerOverflow=on
  Sum1 : Sum  Inputs=+++  SaturateOnIntegerOverflow=on
  Sum2 : Sum  SaturateOnIntegerOverflow=on
  Sum3 : Sum  Inputs=-+  SaturateOnIntegerOverflow=on
  Sum4 : Sum  SaturateOnIntegerOverflow=on
  Sum5 : Sum  SaturateOnIntegerOverflow=on
  Switch : Switch  Criteria=u2 > Threshold
  Switch1 : Switch  Criteria=u2 > Threshold
  Ttask : Gain  Gain=Ts  SaturateOnIntegerOverflow=on  OutDataTypeStr=Inherit: Same as input  ParamDataTypeStr=Inherit: Same as input
  Umrechnung I in Y : Product  SaturateOnIntegerOverflow=on  OutDataTypeStr=Inherit: Same as first input
  Unit Delay : UnitDelay  SampleTime=-1
  Vorsteuerung : Product  SaturateOnIntegerOverflow=on  OutDataTypeStr=Inherit: Same as first input
  Zero : Constant  Value=0
  Zero1 : Constant  Value=0
  i-Delta : Product  SaturateOnIntegerOverflow=on  OutDataTypeStr=Inherit: Same as first input
  p-Anteil : Product  SaturateOnIntegerOverflow=on  OutDataTypeStr=Inherit: Same as first input
  y_req : Outport
  MeasPi : Outport  Port=2
  wires:
  [y_d] -> Bus Creator/6  "y_d"
  kp/1 -> p-Anteil/2
  x_req/1 -> Vorsteuerung/2, [x_act], Sum/1
  yg_limmax/1 -> Subsystem/4(yg_limmax1)
  [y_req] -> Bus Creator/14  "y_req"
  p-Anteil/1 -> [y_p], Sum1/2
  y_des/1 -> Sum3/1, Sum4/1, [y_des]
  Subsystem/1(y_req1) -> Subsystem1/1(y_ref), y_req/1, [y_req]  "y_req"
  Switch1/1 -> [I_1], Sum5/2
  kyi/1 -> Subsystem1/5(kyi1)
  Subsystem1/1(I_k_1) -> Switch1/1
  [y_i] -> Bus Creator/7  "y_i"
  y_max/1 -> Subsystem/2(y_max1), [y_max]
  y_min/1 -> Subsystem/3(y_min1), [y_min]
  x_act/1 -> Dämpfungs- anteil/1, [x_req], Sum/2
  Sum4/1 -> Subsystem/1(x_act1), [y_ref]
  Switch/1 -> Sum4/2
  Umrechnung I in Y/1 -> Sum2/2  "y_i"
  Subsystem/2(ydif_lim) -> Subsystem1/2(ydif_lim)
  [y_max] -> Bus Creator/11  "y_max"
  [y_pdv] -> Bus Creator/8  "y_pdv"
  Sum1/1 -> Sum3/2, [y_pdv], Sum2/1  "y_pdv"
  [y_p] -> Bus Creator/5  "y_p"
  Sum/1 -> p-Anteil/1, [x_e], i-Delta/1
  Vorsteuerung/1 -> [y_v], Sum1/1
  [y_des] -> Bus Creator/13  "y_des"
  Dämpfungs- anteil/1 -> [y_d], Sum1/3
  Sum2/1 -> Switch/1
  [y_v] -> Bus Creator/4  "y_v"
  [I_1] -> Bus Creator/10  "I_1"
  kiy/1 -> Umrechnung I in Y/1
  Sum5/1 -> Unit Delay/1
  kv/1 -> Vorsteuerung/1
  [I] -> Bus Creator/9  "I"
  [x_act] -> Bus Creator/1  "x_act"
  Unit Delay/1 -> Subsystem1/4(I_k), Umrechnung I in Y/2, [I]  "I_k"
  [y_min] -> Bus Creator/12  "y_min"
  [x_e] -> Bus Creator/3  "x_e"
  Ttask/1 -> i-Delta/2
  kd/1 -> Dämpfungs- anteil/2
  ki/1 -> Ttask/1
  [x_req] -> Bus Creator/2  "x_req"
  Sum3/1 -> Subsystem1/3(y_pdv)
  Bus Creator/1 -> MeasPi/1
  [y_ref] -> Bus Creator/15  "y_ref"
  bEnable/1 -> Switch1/2, Switch/2
  Zero/1 -> Switch/3
  Zero1/1 -> Switch1/3
  i-Delta/1 -> [y_i], Sum5/1

== system DIME12_Ctrl_dSpaceHRBMAB/DIME Regler/Controller/Trigger_250us ==
  Counter Limited : simulink/Sources/Counter Limited  uplimit=4  tsamp=-1
  Lookup Table : Lookup_n-D  NumberOfTableDimensions=1  BreakpointsForDimension1=[0,1,2,3,4]  Table=[1,0,0,0,0]  ExtrapMethod=Clip  InputSameDT=on
  trigger : Outport
  wires:
  Counter Limited/1 -> Lookup Table/1
  Lookup Table/1 -> trigger/1

== system DIME12_Ctrl_dSpaceHRBMAB/DIME Regler/Controller/mpsTestMode ==
  note: Integrate the velocity signal to derive electrical position
  Constant6 : Constant  Value=2*pi
  Mod : Math  Operator=mod  SaturateOnIntegerOverflow=on
  PositionIntegrator : Subsystem
  Velocitylimit : Subsystem
  motEleclPosn : Gain  LoadFcn=|  Gain=p
      | if exist('SL_HighlightBlocks', 'file') == 2
      |     if ~SL_HighlightBlocks(gcb, [])
      |         warning(['Unable to set properties for ' gcb])
      |     end
      | end
  mpsTestMaxVelocityDmd : Constant  Value=mpsTestMaxVelocityDmd
  mpsTestVelocityDmd : Constant  Value=mpsTestVelocityDmd
  negLimit : Gain  Gain=-1
  positionIncrement : Gain  Gain=EDC_CURRENT_CONTROL_EXECUTION_PERIOD
  rev2Rad : Gain  Gain=2*pi
  theta : Outport
  wires:
  Constant6/1 -> Mod/2
  rev2Rad/1 -> PositionIntegrator/1(Inc)
  motEleclPosn/1 -> Mod/1  "motEleclPosn"
  PositionIntegrator/1(relMotMeclPosn) -> motEleclPosn/1  "relMotMeclPosn"
  Velocitylimit/1(limdInput) -> positionIncrement/1  "motMeclVelocity"
  mpsTestMaxVelocityDmd/1 -> Velocitylimit/1(UpperLimit), negLimit/1
  mpsTestVelocityDmd/1 -> Velocitylimit/2(unlimdInput)
  Mod/1 -> theta/1
  positionIncrement/1 -> rev2Rad/1
  negLimit/1 -> Velocitylimit/3(LowerLimit)

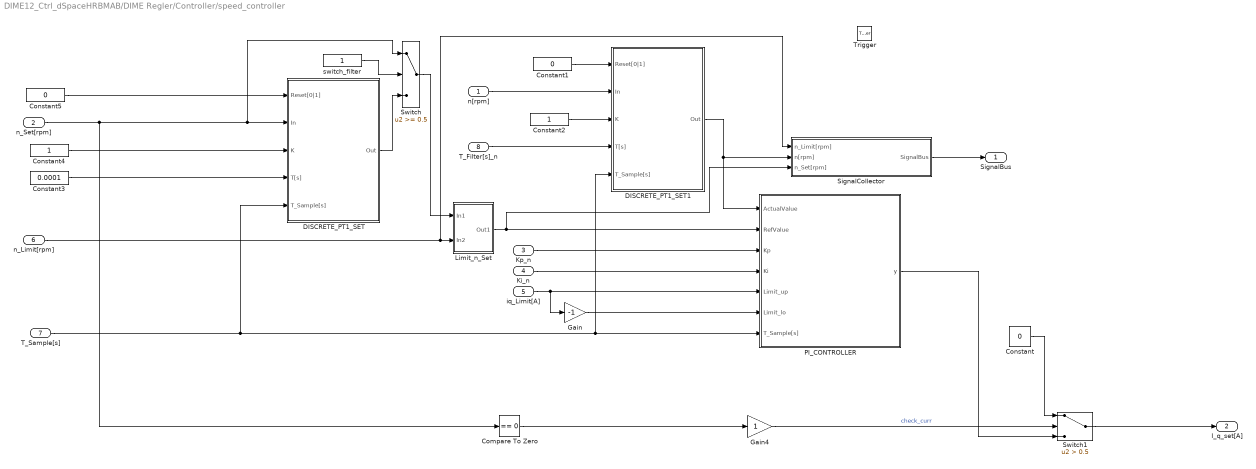
== system DIME12_Ctrl_dSpaceHRBMAB/DIME Regler/Controller/speed_controller ==
  n[rpm] : Inport
  n_Set[rpm] : Inport  Port=2
  Kp_n : Inport  Port=3
  Ki_n : Inport  Port=4
  iq_Limit[A] : Inport  Port=5
  n_Limit[rpm] : Inport  Port=6
  T_Sample[s] : Inport  Port=7
  T_Filter[s]_n : Inport  Port=8
  Trigger : TriggerPort  VariantControl=Variant
  Compare To Zero : simulink/Logic and Bit Operations/Compare To Zero  relop===  OutDataTypeStr=uint8
  Constant : Constant  Value=0
  Constant1 : Constant  Value=0
  Constant2 : Constant
  Constant3 : Constant  Value=0.0001
  Constant4 : Constant
  Constant5 : Constant  Value=0
  DISCRETE_PT1_SET : Subsystem
  DISCRETE_PT1_SET1 : Subsystem
  Gain : Gain  Gain=-1
  Gain4 : Gain
  Limit_n_Set : Subsystem
      mask Display: plot([0.15 0.85],[.5 .5],[.5 .5],[0.05 0.95],0.15+0.7*[0 .25 .75 1],0.05+0.9*[.25 .25 .75 .75]);
  PI_CONTROLLER : Subsystem
  SignalCollector : Subsystem
  Switch : Switch  Threshold=0.5
  Switch1 : Switch  Criteria=u2 > Threshold  Threshold=0.5
  switch_filter : Constant
  SignalBus : Outport
  I_q_set[A] : Outport  Port=2
  wires:
  SignalCollector/1(SignalBus) -> SignalBus/1
  PI_CONTROLLER/1(y) -> Switch1/3
  Kp_n/1 -> PI_CONTROLLER/3(Kp)
  Ki_n/1 -> PI_CONTROLLER/4(Ki)
  iq_Limit[A]/1 -> PI_CONTROLLER/5(Limit_up), Gain/1
  Gain/1 -> PI_CONTROLLER/6(Limit_lo)
  T_Sample[s]/1 -> DISCRETE_PT1_SET1/5(T_Sample[s]), PI_CONTROLLER/7(T_Sample[s]), DISCRETE_PT1_SET/5(T_Sample[s])
  n_Limit[rpm]/1 -> SignalCollector/1(n_Limit[rpm]), Limit_n_Set/2(In2)
  n[rpm]/1 -> DISCRETE_PT1_SET1/2(In)
  Constant1/1 -> DISCRETE_PT1_SET1/1(Reset[0|1])
  Constant2/1 -> DISCRETE_PT1_SET1/3(K)
  T_Filter[s]_n/1 -> DISCRETE_PT1_SET1/4(T[s])
  Limit_n_Set/1(Out1) -> PI_CONTROLLER/2(RefValue), SignalCollector/3(n_Set[rpm])
  DISCRETE_PT1_SET1/1(Out) -> SignalCollector/2(n[rpm]), PI_CONTROLLER/1(ActualValue)
  n_Set[rpm]/1 -> Compare To Zero/1, DISCRETE_PT1_SET/2(In), Switch/1
  Constant3/1 -> DISCRETE_PT1_SET/4(T[s])
  Constant4/1 -> DISCRETE_PT1_SET/3(K)
  Constant5/1 -> DISCRETE_PT1_SET/1(Reset[0|1])
  DISCRETE_PT1_SET/1(Out) -> Switch/3
  Switch/1 -> Limit_n_Set/1(In1)
  switch_filter/1 -> Switch/2
  Compare To Zero/1 -> Gain4/1
  Switch1/1 -> I_q_set[A]/1
  Constant/1 -> Switch1/1
  Gain4/1 -> Switch1/2  "check_curr"

== system DIME12_Ctrl_dSpaceHRBMAB/DIME Regler/Outputs/AKS ==
  Mux1 : Mux  Inputs=3
  U : Constant  Value=0
  V : Constant  Value=0
  W : Constant  Value=0
  DutyCycle : Outport
  wires:
  V/1 -> Mux1/2
  U/1 -> Mux1/1
  W/1 -> Mux1/3
  Mux1/1 -> DutyCycle/1

== system DIME12_Ctrl_dSpaceHRBMAB/DIME Regler/Outputs/Error Protection ==
  In1 : Inport
  In2 : Inport  Port=2
  In3 : Inport  Port=3
  In4 : Inport  Port=4
  In5 : Inport  Port=5
  Logical Operator1 : Logic  Operator=OR  Inputs=4  AllPortsSameDT=off  OutDataTypeStr=boolean
  Terminator1 : Terminator
  current U : Subsystem
  current V : Subsystem
  current W : Subsystem
  speed : Subsystem
  termperature : Subsystem
  Error : Outport
  wires:
  current U/1(Inverter_Current_U_Fault) -> Logical Operator1/1
  In5/1 -> termperature/1(Temperature)
  termperature/1(Inverter_Temp_Fault) -> Logical Operator1/4
  current V/1(Inverter_Current_V_Fault) -> Logical Operator1/2
  In3/1 -> current V/1(Iphase2)
  speed/1(Engine_Speed_Fault) -> Terminator1/1
  current W/1(Inverter_Current_W_Fault) -> Logical Operator1/3
  In1/1 -> speed/1(meclVelocityMAB)
  In2/1 -> current U/1(Iphase1)
  In4/1 -> current W/1(Iphase3)
  Logical Operator1/1 -> Error/1

== system DIME12_Ctrl_dSpaceHRBMAB/DIME Regler/Outputs/SVM ==
  abVoltageDmd : Inport
  Demux : Demux  Outputs=2
  SPACE_VECTOR_MODULATOR : Subsystem
  Valpha1 : Scope
  Vbeta1 : Scope
  voltage transformation inverse clark : Subsystem
  VoltageSynthesizingBus : Outport
  wires:
  voltage transformation inverse clark/1("[3]") -> SPACE_VECTOR_MODULATOR/1(v_Stator[a;b;c][V])
  SPACE_VECTOR_MODULATOR/1(DutyCycle_HSD[a;b;c][0_1]) -> VoltageSynthesizingBus/1
  Demux/2 -> voltage transformation inverse clark/2(beta), Vbeta1/1
  abVoltageDmd/1 -> Demux/1
  Demux/1 -> Valpha1/1, voltage transformation inverse clark/1(alpha)

== system DIME12_Ctrl_dSpaceHRBMAB/DIME Regler/Outputs/SVPWM ==
  U_alpha : Inport
  U_beta : Inport  Port=2
  Calculate Duty Cycles 1 : Subsystem
  Calculate Duty Cycles 2 : Subsystem
  Demux : Demux  Outputs=2
  Demux1 : Demux  Outputs=2
  Sector Select : Subsystem
  Sector Select1 : Subsystem
  reference U* : Subsystem
  reference U*1 : Subsystem
  Duty Cycles 1 : Outport
  Duty Cycles 2 : Outport  Port=2
  wires:
  reference U*/2(angle) -> Calculate Duty Cycles 1/3(angle), Sector Select/1(angle)
  reference U*/1(U*) -> Calculate Duty Cycles 1/1(U*)
  Sector Select/1(Sector) -> Calculate Duty Cycles 1/2(Sector)
  Calculate Duty Cycles 1/1(Duty Cycles) -> Duty Cycles 1/1
  Sector Select1/1(Sector) -> Calculate Duty Cycles 2/2(Sector)
  U_alpha/1 -> Demux/1
  Demux/1 -> reference U*/1(In1)
  U_beta/1 -> Demux1/1
  Demux1/1 -> reference U*/2(In2)
  Demux/2 -> reference U*1/1(In1)
  Demux1/2 -> reference U*1/2(In2)
  reference U*1/2(angle) -> Calculate Duty Cycles 2/3(angle), Sector Select1/1(angle)
  reference U*1/1(U*) -> Calculate Duty Cycles 2/1(U*)
  Calculate Duty Cycles 2/1(Duty Cycles) -> Duty Cycles 2/1

== system DIME12_Ctrl_dSpaceHRBMAB/DIME Regler/dSpace Measurement/Inc Position Input ==
  2PI : Constant  Value=2*pi
  ActivateFilter : Constant  Value=0
  Add : Sum
  AngleOffset_rad : Constant  Value=4.17
  Digital Incremental Encoder In (1) : dsmpblib/Data Inport  Priority=10000
      settings: SourceProductName=dSPACE Model Interface Blockset
  Math Function : Math  Operator=mod  SaturateOnIntegerOverflow=on
  Moving Average : MATLAB Function  TreatAsAtomicUnit=on
  Omega_rpsUnfilterd : Scope
  Switch9 : Switch  Criteria=u2 > Threshold
  bool2double : DataTypeConversion
  degree per sec to rps : Gain  Gain=1/(360)
  inc_valid : Scope
  motMecPosn : Scope
  posnScalingMAB : Gain  Gain=pi/180
  Incremental_Derivative_Velocity[Rps] : Outport
  motEleclPosn : Outport  Port=2
  wires:
  Digital Incremental Encoder In (1)/3 -> bool2double/1
  Digital Incremental Encoder In (1)/1 -> degree per sec to rps/1
  bool2double/1 -> inc_valid/1  "inc_valid"
  AngleOffset_rad/1 -> Add/1
  Add/1 -> Math Function/1
  posnScalingMAB/1 -> Add/2
  2PI/1 -> Math Function/2
  Digital Incremental Encoder In (1)/2 -> posnScalingMAB/1, motMecPosn/1
  Math Function/1 -> motEleclPosn/1
  ActivateFilter/1 -> Switch9/2
  Moving Average/1(ymean) -> Switch9/1
  degree per sec to rps/1 -> Omega_rpsUnfilterd/1, Switch9/3, Moving Average/1(y)
  Switch9/1 -> Incremental_Derivative_Velocity[Rps]/1

== system DIME12_Ctrl_dSpaceHRBMAB/DIME Regler/Controller/Num_Differentiatior_ControllerTask_Ts/Int ==
  i_d_p : Inport
  Gain1 : Gain
  Sum4 : Sum  Inputs=|++
  Ts_is_1_by_40kHz : Gain  Gain=Ts
  Unit Delay1 : UnitDelay  SampleTime=-1
  i_d : Outport  VectorParamsAs1DForOutWhenUnconnected=on
  wires:
  Gain1/1 -> Unit Delay1/1
  Sum4/1 -> Gain1/1
  Ts_is_1_by_40kHz/1 -> Sum4/1
  Unit Delay1/1 -> i_d/1, Sum4/2  "i_d"
  i_d_p/1 -> Ts_is_1_by_40kHz/1

== system DIME12_Ctrl_dSpaceHRBMAB/DIME Regler/Controller/Num_Differentiatior_ControllerTask_Ts/Int1 ==
  i_q_p : Inport
  Gain1 : Gain
  Sum4 : Sum  Inputs=|++
  Ts_is_1_by_40kHz : Gain  Gain=Ts
  Unit Delay1 : UnitDelay  SampleTime=-1
  i_q : Outport  VectorParamsAs1DForOutWhenUnconnected=on
  wires:
  i_q_p/1 -> Ts_is_1_by_40kHz/1
  Unit Delay1/1 -> Sum4/2, i_q/1  "i_d"
  Ts_is_1_by_40kHz/1 -> Sum4/1
  Sum4/1 -> Gain1/1
  Gain1/1 -> Unit Delay1/1

== system DIME12_Ctrl_dSpaceHRBMAB/DIME Regler/Controller/Subsystem1/Subsystem ==
  x_act1 : Inport
  y_max1 : Inport  Port=2
  y_min1 : Inport  Port=3
  yg_limmax1 : Inport  Port=4
  1/Ttask : Gain  Gain=Ts  SaturateOnIntegerOverflow=on  OutDataTypeStr=Inherit: Same as input  ParamDataTypeStr=Inherit: Same as input
  Abs : Abs
  Delay by Ta : UnitDelay  SampleTime=-1
  Divide2 : Product  Inputs=**
  Maximum : MinMax  Inputs=2  SaturateOnIntegerOverflow=on  InputSameDT=on
  Min1 : MinMax  Inputs=2  SaturateOnIntegerOverflow=on  InputSameDT=on
  Minimum : MinMax  Function=max  Inputs=2  SaturateOnIntegerOverflow=on  InputSameDT=on
  Sign : Signum
  Sum6 : Sum  Inputs=+-  SaturateOnIntegerOverflow=on
  Sum7 : Sum  Inputs=|+-  SaturateOnIntegerOverflow=on
  Sum8 : Sum  Inputs=|++  SaturateOnIntegerOverflow=on
  y_req1 : Outport
  ydif_lim : Outport  Port=2
  wires:
  y_max1/1 -> Maximum/1
  x_act1/1 -> Sum7/1
  Minimum/1 -> y_req1/1, Sum6/2, Delay by Ta/1
  Sum7/1 -> Sign/1, Abs/1
  Abs/1 -> Min1/2
  Maximum/1 -> Minimum/1
  Delay by Ta/1 -> Sum8/2, Sum7/2
  1/Ttask/1 -> Min1/1
  Sign/1 -> Divide2/2
  yg_limmax1/1 -> 1/Ttask/1
  Min1/1 -> Divide2/1
  y_min1/1 -> Minimum/2
  Sum8/1 -> Sum6/1, Maximum/2
  Divide2/1 -> Sum8/1
  Sum6/1 -> ydif_lim/1

== system DIME12_Ctrl_dSpaceHRBMAB/DIME Regler/Controller/Subsystem1/Subsystem1 ==
  y_ref : Inport
  ydif_lim : Inport  Port=2
  y_pdv : Inport  Port=3
  I_k : Inport  Port=4
  kyi1 : Inport  Port=5
  Max1 : MinMax  Function=max  Inputs=2  SaturateOnIntegerOverflow=on  InputSameDT=on
  Min3 : MinMax  Inputs=2  SaturateOnIntegerOverflow=on  InputSameDT=on
  Sum8 : Sum  Inputs=-+
  Sum9 : Sum  Inputs=-+
  Switch2 : Switch
  Switch3 : Switch  Criteria=u2 ~= 0
  Umrechnung Wertebereich Y in I : Product  SaturateOnIntegerOverflow=on  OutDataTypeStr=Inherit: Same as first input
  zero1 : Constant  Value=0
  I_k_1 : Outport
  wires:
  Max1/1 -> Switch2/1
  ydif_lim/1 -> Switch2/2, Switch3/2
  y_pdv/1 -> Sum8/1, Sum9/1
  y_ref/1 -> Sum8/2, Sum9/2
  I_k/1 -> Switch3/3
  Sum8/1 -> Max1/1
  Switch3/1 -> I_k_1/1
  Umrechnung Wertebereich Y in I/1 -> Switch3/1
  Switch2/1 -> Umrechnung Wertebereich Y in I/2
  Sum9/1 -> Min3/2
  kyi1/1 -> Umrechnung Wertebereich Y in I/1
  Min3/1 -> Switch2/3
  zero1/1 -> Min3/1, Max1/2

== system DIME12_Ctrl_dSpaceHRBMAB/DIME Regler/Controller/Subsystem2/Subsystem ==
  x_act1 : Inport
  y_max1 : Inport  Port=2
  y_min1 : Inport  Port=3
  yg_limmax1 : Inport  Port=4
  1/Ttask : Gain  Gain=Ts  SaturateOnIntegerOverflow=on  OutDataTypeStr=Inherit: Same as input  ParamDataTypeStr=Inherit: Same as input
  Abs : Abs
  Delay by Ta : UnitDelay  SampleTime=-1
  Divide2 : Product  Inputs=**
  Maximum : MinMax  Inputs=2  SaturateOnIntegerOverflow=on  InputSameDT=on
  Min1 : MinMax  Inputs=2  SaturateOnIntegerOverflow=on  InputSameDT=on
  Minimum : MinMax  Function=max  Inputs=2  SaturateOnIntegerOverflow=on  InputSameDT=on
  Sign : Signum
  Sum6 : Sum  Inputs=+-  SaturateOnIntegerOverflow=on
  Sum7 : Sum  Inputs=|+-  SaturateOnIntegerOverflow=on
  Sum8 : Sum  Inputs=|++  SaturateOnIntegerOverflow=on
  y_req1 : Outport
  ydif_lim : Outport  Port=2
  wires:
  y_max1/1 -> Maximum/1
  x_act1/1 -> Sum7/1
  Minimum/1 -> y_req1/1, Sum6/2, Delay by Ta/1
  Sum7/1 -> Sign/1, Abs/1
  Abs/1 -> Min1/2
  Maximum/1 -> Minimum/1
  Delay by Ta/1 -> Sum8/2, Sum7/2
  1/Ttask/1 -> Min1/1
  Sign/1 -> Divide2/2
  yg_limmax1/1 -> 1/Ttask/1
  Min1/1 -> Divide2/1
  y_min1/1 -> Minimum/2
  Sum8/1 -> Sum6/1, Maximum/2
  Divide2/1 -> Sum8/1
  Sum6/1 -> ydif_lim/1

== system DIME12_Ctrl_dSpaceHRBMAB/DIME Regler/Controller/Subsystem2/Subsystem1 ==
  y_ref : Inport
  ydif_lim : Inport  Port=2
  y_pdv : Inport  Port=3
  I_k : Inport  Port=4
  kyi1 : Inport  Port=5
  Max1 : MinMax  Function=max  Inputs=2  SaturateOnIntegerOverflow=on  InputSameDT=on
  Min3 : MinMax  Inputs=2  SaturateOnIntegerOverflow=on  InputSameDT=on
  Sum8 : Sum  Inputs=-+
  Sum9 : Sum  Inputs=-+
  Switch2 : Switch
  Switch3 : Switch  Criteria=u2 ~= 0
  Umrechnung Wertebereich Y in I : Product  SaturateOnIntegerOverflow=on  OutDataTypeStr=Inherit: Same as first input
  zero1 : Constant  Value=0
  I_k_1 : Outport
  wires:
  Max1/1 -> Switch2/1
  ydif_lim/1 -> Switch2/2, Switch3/2
  y_pdv/1 -> Sum8/1, Sum9/1
  y_ref/1 -> Sum8/2, Sum9/2
  I_k/1 -> Switch3/3
  Sum8/1 -> Max1/1
  Switch3/1 -> I_k_1/1
  Umrechnung Wertebereich Y in I/1 -> Switch3/1
  Switch2/1 -> Umrechnung Wertebereich Y in I/2
  Sum9/1 -> Min3/2
  kyi1/1 -> Umrechnung Wertebereich Y in I/1
  Min3/1 -> Switch2/3
  zero1/1 -> Min3/1, Max1/2

== system DIME12_Ctrl_dSpaceHRBMAB/DIME Regler/Controller/mpsTestMode/PositionIntegrator ==
  Inc : Inport
  Constant : Constant  Value=2*pi
  Mod : Math  Operator=mod  SaturateOnIntegerOverflow=on
  motMeclPosn : Sum  LoadFcn=|
      | if exist('SL_HighlightBlocks', 'file') == 2
      |     if ~SL_HighlightBlocks(gcb, [])
      |         warning(['Unable to set properties for ' gcb])
      |     end
      | end
  posnIntegral : UnitDelay  SampleTime=-1
      settings: AttributesFormatString=Initial Condition = %<InitialCondition>
  relMotMeclPosn : Outport
  wires:
  posnIntegral/1 -> motMeclPosn/2
  Inc/1 -> motMeclPosn/1
  motMeclPosn/1 -> Mod/1
  Constant/1 -> Mod/2
  Mod/1 -> posnIntegral/1, relMotMeclPosn/1

== system DIME12_Ctrl_dSpaceHRBMAB/DIME Regler/Controller/mpsTestMode/Velocitylimit ==
  UpperLimit : Inport
  unlimdInput : Inport  Port=2
  LowerLimit : Inport  Port=3
  If : If  NumInputs=3  IfExpression=u1 > u2  ElseIfExpressions=u1 < u3
  LimitMerge : Merge  Inputs=3  InitialOutput=0
  Subsystem : Subsystem
  Subsystem1 : Subsystem
  Subsystem2 : Subsystem
  limdInput : Outport
  wires:
  Subsystem2/1(limdInput) -> LimitMerge/1
  LimitMerge/1 -> limdInput/1
  UpperLimit/1 -> Subsystem2/1(UpperLimit), If/2
  unlimdInput/1 -> Subsystem/1(unlimdInput), If/1
  If/1 -> Subsystem2/Action
  If/2 -> Subsystem1/Action
  LowerLimit/1 -> Subsystem1/1(LowerLimit), If/3
  Subsystem1/1(limdInput) -> LimitMerge/2
  If/3 -> Subsystem/Action
  Subsystem/1(limdInput) -> LimitMerge/3
